simulink model "Position"  (R2016b)
settings: Solver=ode2  StartTime=0.0  StopTime=10.0  FixedStep=sample_time  RelTol=1e-3  EnableMultiTasking=on
InitFcn:
  | Parameters_physical_tiltrotor
  | Parameters_controllers_tiltrotor
undefined symbols (not defined in the file): ALT_N, gravity, KB_U, KB_V, KB_X, KB_Y, KB_Z, KD_U, KD_V, KD_X, KD_Y, KD_Z, KI_U, KI_V, KI_X, KI_Y, KI_Z, KP_U, KP_V, KP_X, KP_Y, KP_Z, mass, MAX_DELTA_THRUST, MAX_U, MAX_V, MAX_VEL, MIN_DELTA_THRUST, MIN_U, MIN_V, MIN_VEL, POS_N, VEL_N
libraries: simulink x5
settings Model: Creator=pela  LastModifiedBy=Mattia
settings DataIOCC: LimitDataPoints=on  SaveFormat=Array
settings OptimizationCC: LifeSpan=inf
settings DebuggingCC: SFUnexpectedBacktrackingDiag=warning  SFNoUnconditionalDefaultTransitionDiag=warning  SFExecutionAtInitializationDiag=none
settings HardwareCC: ProdBitPerPointer=32  ProdBitPerSizeT=32  ProdBitPerPtrDiffT=32  ProdLargestAtomicInteger=Long  ProdLargestAtomicFloat=Double  ProdIntDivRoundTo=Undefined  ProdWordSize=32  ProdHWDeviceType=ARM Compatible->ARM Cortex
settings ModelReferenceCC: PropagateSignalLabelsOutOfModel=off
settings RTWCC: GenCodeOnly=on  GenerateReport=on  Toolchain=GNU gcc/g++ v4.4.x | gmake (64-bit Linux)  BuildConfiguration=Faster Runs  LaunchReport=on  TargetLang=C++
settings GRTTargetCC: TargetLangStandard=C89/C90 (ANSI)  GeneratePreprocessorConditionals=Disable all  MatFileLogging=off  MultiInstanceERTCode=on  CodeInterfacePackaging=C++ class  SupportNonFinite=off
settings ConfigComp: CovMetricSettings=dw  CovHtmlReporting=on  CovSaveCumulativeToWorkspaceVar=on  CovSaveSingleToWorkspaceVar=on  CovExternalEMLEnable=off

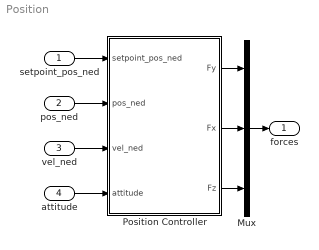
== system Position ==
  setpoint_pos_ned : Inport  PortDimensions=3
  pos_ned : Inport  Port=2  PortDimensions=3
  vel_ned : Inport  Port=3  PortDimensions=3
  attitude : Inport  Port=4
  Mux : Mux  Inputs=3
  Position Controller : Subsystem
  forces : Outport
  wires:
  setpoint_pos_ned/1 -> Position Controller/1(setpoint_pos_ned)
  attitude/1 -> Position Controller/4(attitude)
  vel_ned/1 -> Position Controller/3(vel_ned)
  pos_ned/1 -> Position Controller/2(pos_ned)
  Position Controller/2(Fx) -> Mux/2
  Mux/1 -> forces/1
  Position Controller/1(Fy) -> Mux/1
  Position Controller/3(Fz) -> Mux/3

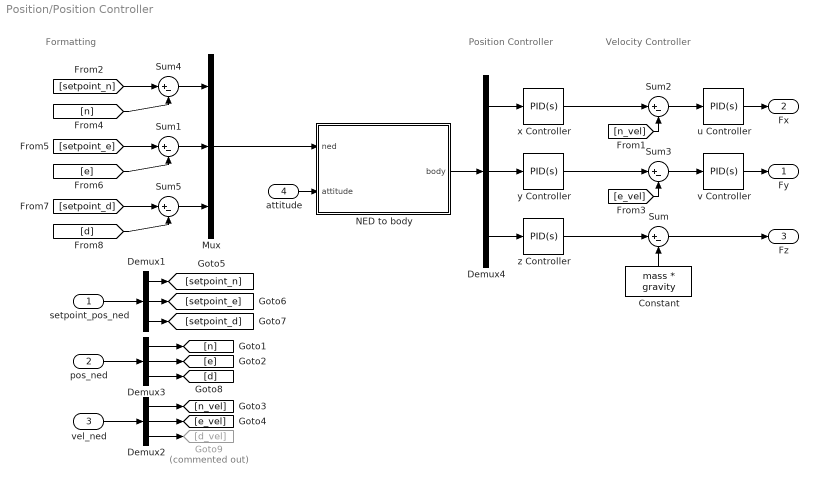
== system Position/Position Controller ==
  note: Formatting
  note: Velocity Controller
  note: Position Controller
  setpoint_pos_ned : Inport  PortDimensions=3
  pos_ned : Inport  Port=2  PortDimensions=3
  vel_ned : Inport  Port=3
  attitude : Inport  Port=4  PortDimensions=3
  Constant : Constant  Value=mass * gravity
  Demux{1..4} (4 alike) : Demux  Outputs=3
  Goto9 : Goto  Commented=on  GotoTag=d_vel
  Mux : Mux  Inputs=3
  NED to body : MATLAB Function  TreatAsAtomicUnit=on
  Sum{,1..5} (6 alike) : Sum  Inputs=|+-
  u Controller : simulink/Continuous/PID Controller  Controller=PID  TimeDomain=Continuous-time  SampleTime=-1  IntegratorMethod=Forward Euler  FilterMethod=Trapezoidal  Form=Parallel  UseFilter=on  ControllerParametersSource=internal  P=KP_U  I=KI_U  D=KD_U  N=VEL_N  InitialConditionSource=internal  InitialConditionForIntegrator=0  InitialConditionForFilter=0  ExternalReset=none  LimitOutput=on  UpperSaturationLimit=MAX_U  LowerSaturationLimit=MIN_U  LinearizeAsGain=on  AntiWindupMode=back-calculation  Kb=KB_U  TrackingMode=off  Kt=1  PParamMin=[]  PParamMax=[]  IParamMin=[]  IParamMax=[]  DParamMin=[]  DParamMax=[]  NParamMin=[]  NParamMax=[]  KbParamMin=[]  KbParamMax=[]  KtParamMin=[]  KtParamMax=[]  POutMin=[]  POutMax=[]  IOutMin=[]  IOutMax=[]  DOutMin=[]  DOutMax=[]  NOutMin=[]  NOutMax=[]  KbOutMin=[]  KbOutMax=[]  KtOutMin=[]  KtOutMax=[]  IntegratorOutMin=[]  IntegratorOutMax=[]  FilterOutMin=[]  FilterOutMax=[]  SumOutMin=[]  SumOutMax=[]  SumI1OutMin=[]  SumI1OutMax=[]  SumI2OutMin=[]  SumI2OutMax=[]  SumI3OutMin=[]  SumI3OutMax=[]  SumDOutMin=[]  SumDOutMax=[]  SaturationOutMin=[]  SaturationOutMax=[]  IntegratorContinuousStateAttributes=''  IntegratorStateMustResolveToSignalObject=off  IntegratorRTWStateStorageClass=Auto  FilterContinuousStateAttributes=''  FilterStateMustResolveToSignalObject=off  FilterRTWStateStorageClass=Auto  DifferentiatorICPrevScaledInput=0  DifferentiatorOutMin=[]  DifferentiatorOutMax=[]
  v Controller : simulink/Continuous/PID Controller  Controller=PID  TimeDomain=Continuous-time  SampleTime=-1  IntegratorMethod=Forward Euler  FilterMethod=Trapezoidal  Form=Parallel  UseFilter=on  ControllerParametersSource=internal  P=KP_V  I=KI_V  D=KD_V  N=VEL_N  InitialConditionSource=internal  InitialConditionForIntegrator=0  InitialConditionForFilter=0  ExternalReset=none  LimitOutput=on  UpperSaturationLimit=MAX_V  LowerSaturationLimit=MIN_V  LinearizeAsGain=on  AntiWindupMode=back-calculation  Kb=KB_V  TrackingMode=off  Kt=1  PParamMin=[]  PParamMax=[]  IParamMin=[]  IParamMax=[]  DParamMin=[]  DParamMax=[]  NParamMin=[]  NParamMax=[]  KbParamMin=[]  KbParamMax=[]  KtParamMin=[]  KtParamMax=[]  POutMin=[]  POutMax=[]  IOutMin=[]  IOutMax=[]  DOutMin=[]  DOutMax=[]  NOutMin=[]  NOutMax=[]  KbOutMin=[]  KbOutMax=[]  KtOutMin=[]  KtOutMax=[]  IntegratorOutMin=[]  IntegratorOutMax=[]  FilterOutMin=[]  FilterOutMax=[]  SumOutMin=[]  SumOutMax=[]  SumI1OutMin=[]  SumI1OutMax=[]  SumI2OutMin=[]  SumI2OutMax=[]  SumI3OutMin=[]  SumI3OutMax=[]  SumDOutMin=[]  SumDOutMax=[]  SaturationOutMin=[]  SaturationOutMax=[]  IntegratorContinuousStateAttributes=''  IntegratorStateMustResolveToSignalObject=off  IntegratorRTWStateStorageClass=Auto  FilterContinuousStateAttributes=''  FilterStateMustResolveToSignalObject=off  FilterRTWStateStorageClass=Auto  DifferentiatorICPrevScaledInput=0  DifferentiatorOutMin=[]  DifferentiatorOutMax=[]
  x Controller : simulink/Continuous/PID Controller  Controller=PID  TimeDomain=Continuous-time  SampleTime=-1  IntegratorMethod=Forward Euler  FilterMethod=Trapezoidal  Form=Parallel  UseFilter=on  ControllerParametersSource=internal  P=KP_X  I=KI_X  D=KD_X  N=POS_N  InitialConditionSource=internal  InitialConditionForIntegrator=0  InitialConditionForFilter=0  ExternalReset=none  LimitOutput=on  UpperSaturationLimit=MAX_VEL  LowerSaturationLimit=MIN_VEL  LinearizeAsGain=on  AntiWindupMode=back-calculation  Kb=KB_X  TrackingMode=off  Kt=1  PParamMin=[]  PParamMax=[]  IParamMin=[]  IParamMax=[]  DParamMin=[]  DParamMax=[]  NParamMin=[]  NParamMax=[]  KbParamMin=[]  KbParamMax=[]  KtParamMin=[]  KtParamMax=[]  POutMin=[]  POutMax=[]  IOutMin=[]  IOutMax=[]  DOutMin=[]  DOutMax=[]  NOutMin=[]  NOutMax=[]  KbOutMin=[]  KbOutMax=[]  KtOutMin=[]  KtOutMax=[]  IntegratorOutMin=[]  IntegratorOutMax=[]  FilterOutMin=[]  FilterOutMax=[]  SumOutMin=[]  SumOutMax=[]  SumI1OutMin=[]  SumI1OutMax=[]  SumI2OutMin=[]  SumI2OutMax=[]  SumI3OutMin=[]  SumI3OutMax=[]  SumDOutMin=[]  SumDOutMax=[]  SaturationOutMin=[]  SaturationOutMax=[]  IntegratorContinuousStateAttributes=''  IntegratorStateMustResolveToSignalObject=off  IntegratorRTWStateStorageClass=Auto  FilterContinuousStateAttributes=''  FilterStateMustResolveToSignalObject=off  FilterRTWStateStorageClass=Auto  DifferentiatorICPrevScaledInput=0  DifferentiatorOutMin=[]  DifferentiatorOutMax=[]
  y Controller : simulink/Continuous/PID Controller  Controller=PID  TimeDomain=Continuous-time  SampleTime=-1  IntegratorMethod=Forward Euler  FilterMethod=Trapezoidal  Form=Parallel  UseFilter=on  ControllerParametersSource=internal  P=KP_Y  I=KI_Y  D=KD_Y  N=POS_N  InitialConditionSource=internal  InitialConditionForIntegrator=0  InitialConditionForFilter=0  ExternalReset=none  LimitOutput=on  UpperSaturationLimit=MAX_VEL  LowerSaturationLimit=MIN_VEL  LinearizeAsGain=on  AntiWindupMode=back-calculation  Kb=KB_Y  TrackingMode=off  Kt=1  PParamMin=[]  PParamMax=[]  IParamMin=[]  IParamMax=[]  DParamMin=[]  DParamMax=[]  NParamMin=[]  NParamMax=[]  KbParamMin=[]  KbParamMax=[]  KtParamMin=[]  KtParamMax=[]  POutMin=[]  POutMax=[]  IOutMin=[]  IOutMax=[]  DOutMin=[]  DOutMax=[]  NOutMin=[]  NOutMax=[]  KbOutMin=[]  KbOutMax=[]  KtOutMin=[]  KtOutMax=[]  IntegratorOutMin=[]  IntegratorOutMax=[]  FilterOutMin=[]  FilterOutMax=[]  SumOutMin=[]  SumOutMax=[]  SumI1OutMin=[]  SumI1OutMax=[]  SumI2OutMin=[]  SumI2OutMax=[]  SumI3OutMin=[]  SumI3OutMax=[]  SumDOutMin=[]  SumDOutMax=[]  SaturationOutMin=[]  SaturationOutMax=[]  IntegratorContinuousStateAttributes=''  IntegratorStateMustResolveToSignalObject=off  IntegratorRTWStateStorageClass=Auto  FilterContinuousStateAttributes=''  FilterStateMustResolveToSignalObject=off  FilterRTWStateStorageClass=Auto  DifferentiatorICPrevScaledInput=0  DifferentiatorOutMin=[]  DifferentiatorOutMax=[]
  z Controller : simulink/Continuous/PID Controller  Controller=PID  TimeDomain=Continuous-time  SampleTime=-1  IntegratorMethod=Forward Euler  FilterMethod=Trapezoidal  Form=Parallel  UseFilter=on  ControllerParametersSource=internal  P=KP_Z  I=KI_Z  D=KD_Z  N=ALT_N  InitialConditionSource=internal  InitialConditionForIntegrator=0  InitialConditionForFilter=0  ExternalReset=none  LimitOutput=on  UpperSaturationLimit=MAX_DELTA_THRUST  LowerSaturationLimit=MIN_DELTA_THRUST  LinearizeAsGain=on  AntiWindupMode=back-calculation  Kb=KB_Z  TrackingMode=off  Kt=1  PParamMin=[]  PParamMax=[]  IParamMin=[]  IParamMax=[]  DParamMin=[]  DParamMax=[]  NParamMin=[]  NParamMax=[]  KbParamMin=[]  KbParamMax=[]  KtParamMin=[]  KtParamMax=[]  POutMin=[]  POutMax=[]  IOutMin=[]  IOutMax=[]  DOutMin=[]  DOutMax=[]  NOutMin=[]  NOutMax=[]  KbOutMin=[]  KbOutMax=[]  KtOutMin=[]  KtOutMax=[]  IntegratorOutMin=[]  IntegratorOutMax=[]  FilterOutMin=[]  FilterOutMax=[]  SumOutMin=[]  SumOutMax=[]  SumI1OutMin=[]  SumI1OutMax=[]  SumI2OutMin=[]  SumI2OutMax=[]  SumI3OutMin=[]  SumI3OutMax=[]  SumDOutMin=[]  SumDOutMax=[]  SaturationOutMin=[]  SaturationOutMax=[]  IntegratorContinuousStateAttributes=''  IntegratorStateMustResolveToSignalObject=off  IntegratorRTWStateStorageClass=Auto  FilterContinuousStateAttributes=''  FilterStateMustResolveToSignalObject=off  FilterRTWStateStorageClass=Auto  DifferentiatorICPrevScaledInput=0  DifferentiatorOutMin=[]  DifferentiatorOutMax=[]
  Fy : Outport  PortDimensions=1
  Fx : Outport  Port=2  PortDimensions=1
  Fz : Outport  Port=3
  wires:
  v Controller/1 -> Fy/1
  pos_ned/1 -> Demux3/1
  Demux2/1 -> [n_vel]
  Demux2/2 -> [e_vel]
  vel_ned/1 -> Demux2/1
  u Controller/1 -> Fx/1
  setpoint_pos_ned/1 -> Demux1/1
  Demux3/1 -> [n]
  Demux3/2 -> [e]
  Demux1/1 -> [setpoint_n]
  Demux1/2 -> [setpoint_e]
  [setpoint_n] -> Sum4/1
  [n] -> Sum4/2
  [setpoint_e] -> Sum1/1
  Sum2/1 -> u Controller/1
  Sum3/1 -> v Controller/1
  x Controller/1 -> Sum2/1
  [n_vel] -> Sum2/2
  y Controller/1 -> Sum3/1
  [e_vel] -> Sum3/2
  [e] -> Sum1/2
  Demux1/3 -> [setpoint_d]
  Demux3/3 -> [d]
  Demux2/3 -> Goto9/1
  [d] -> Sum5/2
  [setpoint_d] -> Sum5/1
  Constant/1 -> Sum/2
  z Controller/1 -> Sum/1
  Sum/1 -> Fz/1
  attitude/1 -> NED to body/2(attitude)
  Sum4/1 -> Mux/1
  Sum1/1 -> Mux/2
  Sum5/1 -> Mux/3
  Mux/1 -> NED to body/1(ned)
  NED to body/1(body) -> Demux4/1
  Demux4/3 -> z Controller/1
  Demux4/2 -> y Controller/1
  Demux4/1 -> x Controller/1

== matlab function Position/Position Controller/NED to body ==
  data: ned input; attitude input; body output
function body  = ned2body( ned, attitude )

phi = 0;
theta = 0;
psi = attitude(3);

Sphi = sin(phi);
Cphi = cos(phi);
Stheta = sin(theta);
Ctheta = cos(theta);
Spsi = sin(psi);
Cpsi = cos(psi);

ned2body = [                 Ctheta*Cpsi,                  Ctheta*Spsi,     -Stheta ;
            Sphi*Stheta*Cpsi - Cphi*Spsi, Sphi*Stheta*Spsi + Cphi*Cpsi, Sphi*Ctheta ;
            Cphi*Stheta*Cpsi + Sphi*Spsi, Cphi*Stheta*Spsi - Sphi*Cpsi, Cphi*Ctheta];

body = ned2body * ned;
